simulink model "aplusbplusc"  (R2024a)
settings: Solver=VariableStepAuto  StartTime=0.0  StopTime=10.0  RelTol=1e-3
settings Model: Creator=Lenovo  LastModifiedBy=Lenovo

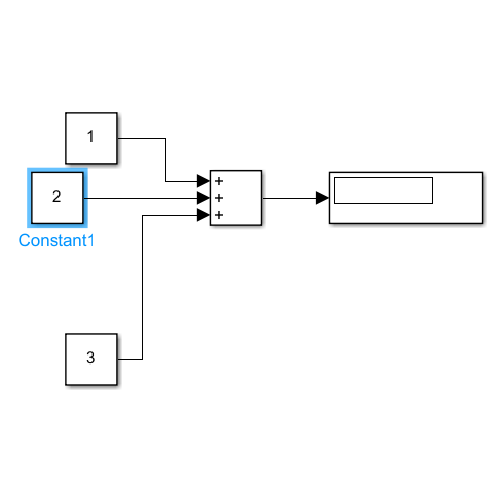
[thumbnail: Simulink's stored preview of the top-level diagram]
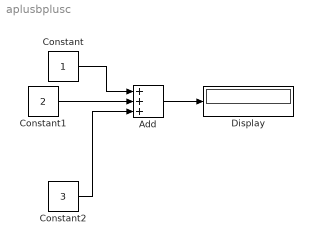
== system aplusbplusc ==
  Add : Sum  Inputs=+++
  Constant : Constant
  Constant1 : Constant  Value=2
  Constant2 : Constant  Value=3
  Display : Display
  wires:
  Constant/1 -> Add/1
  Constant1/1 -> Add/2
  Add/1 -> Display/1
  Constant2/1 -> Add/3
